simulink model "air_part1_python"  (R2022b)
settings: Solver=FixedStepAuto  StartTime=0.0  StopTime=35  FixedStep=0.00005  MinStep=1e-3  RelTol=1e-3
libraries: slrealtimeseriallib x7, simulink x2, instrumentlib x2, etargetslib x1
settings Model: Creator=riku3  LastModifiedBy=riku3
settings SolverCC: ZeroCrossControl=DisableAll  ZeroCrossAlgorithm=Adaptive
settings DebuggingCC: IgnoredZcDiagnostic=none  UnconnectedInputMsg=warning  UnconnectedOutputMsg=warning  UnconnectedLineMsg=warning
settings ModelReferenceCC: EnableRefExpFcnMdlSchedulingChecks=on
settings RTWCC: DLArmComputeVersion=19.05

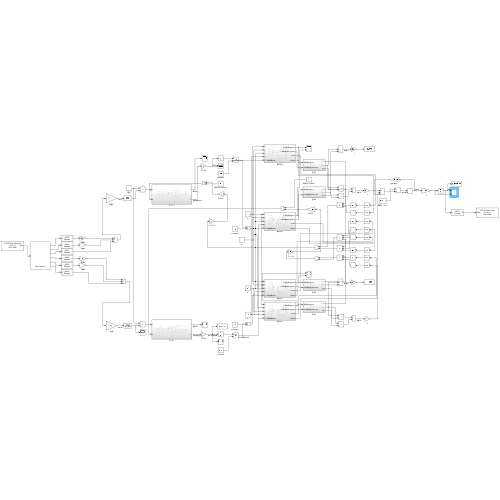
[thumbnail: Simulink's stored preview of the top-level diagram]
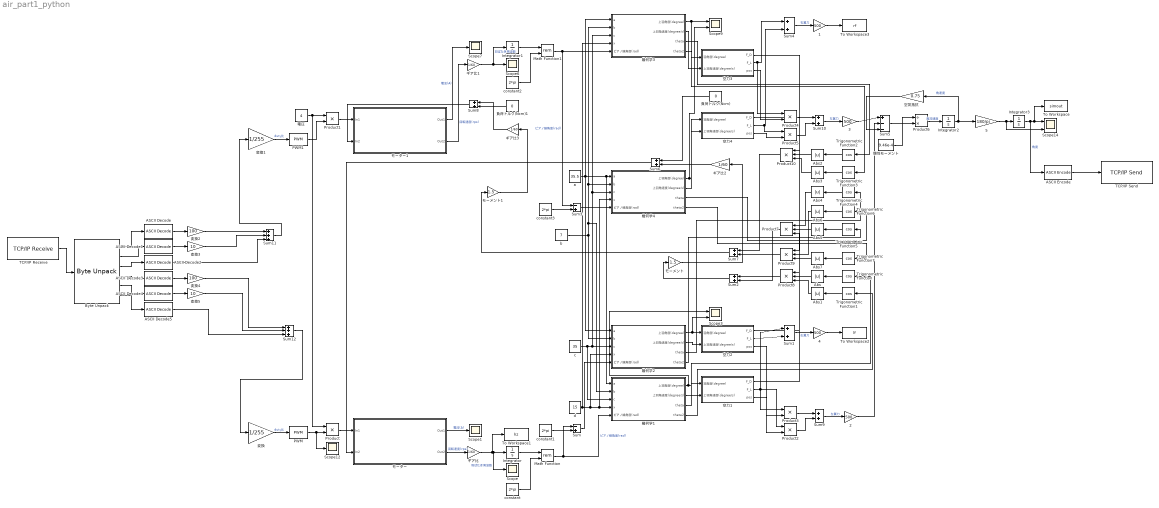
== system air_part1_python ==
  {1..4} (4 alike) : Gain  Gain=500
  5 : Gain  Gain=180/pi
  ASCII Decode{,1..5} (6 alike) : slrealtimeseriallib/ASCII Decode  format=%d\r  nvars=1  vartypes={ }
  ASCII Encode : slrealtimeseriallib/ASCII Encode  format=%d\r  nvars=1  maxlength=128  vartypes={ 'double' }
  Abs{,1..7} (8 alike) : Abs  SaturateOnIntegerOverflow=off
  Byte Unpack : etargetslib/Byte Unpack  dimensions={[1],[1],[1],[1],[1],[1]}  datatypes={'uint8','uint8','uint8','uint8','uint8','uint8'}  byteAlign=1
  Integrator : Integrator
  Integrator1 : Integrator
  Integrator2 : Integrator
  Integrator3 : Integrator  InitialCondition=-90
  Math Function : Math  Operator=rem
  Math Function1 : Math  Operator=rem
  PWM : simulink/Discontinuities/PWM  DisableCoverage=on  Period=0.001  InitialDelay=0  DisallowZeroDutyCycle=off  RunAtFixedTimeIntervals=on  SampleTime=0.00005
  PWM1 : simulink/Discontinuities/PWM  DisableCoverage=on  Period=0.001  InitialDelay=0  DisallowZeroDutyCycle=off  RunAtFixedTimeIntervals=on  SampleTime=0.00005
  Product : Product  Inputs=**
  Product1 : Product  Inputs=**
  Product{7..10} (4 alike) : Product  Inputs=3
  Product{2..5} (4 alike) : Product
  Product6 : Product  Inputs=/*
  Scope{,1,6..7,12} (5 alike) : Scope
  Scope14 : Scope  NumInputPorts=2
  Scope3 : Scope  NumInputPorts=2
  Scope9 : Scope  NumInputPorts=2
  Sum : Sum  Inputs=-+
  Sum1 : Sum  Inputs=|++
  Sum{2,6..10} (6 alike) : Sum
  Sum11 : Sum  Inputs=+++
  Sum12 : Sum  Inputs=+++
  Sum3 : Sum  Inputs=-+
  Sum4 : Sum  Inputs=|++
  Sum5 : Sum  Inputs=|+--
  TCP/IP Receive : instrumentlib/TCP//IP Receive  Host=127.0.0.1  Port=9999  DataSize=[6]  DataType=uint8  ASCIIFormatting=%d  Terminator=LF  CustomTerminator=10  ByteOrder=big-endian  EnableBlockingMode=on  Timeout=10  SampleTime=0.04  SimulateUsing=Interpreted execution
  TCP/IP Send : instrumentlib/TCP//IP Send  Host=127.0.0.1  Port=9999  ByteOrder=big-endian  EnableBlockingMode=on  Timeout=10  TransferDelay=on  SimulateUsing=Interpreted execution
  To Workspace : ToWorkspace  VariableName=simout  SaveFormat=Timeseries  SampleTime=-1
  To Workspace1 : ToWorkspace  VariableName=hz  SaveFormat=Timeseries  SampleTime=-1
  To Workspace2 : ToWorkspace  VariableName=lf  SaveFormat=Timeseries  SampleTime=-1
  To Workspace3 : ToWorkspace  VariableName=rf  SaveFormat=Timeseries  SampleTime=-1
  Trigonometric Function{,1..7} (8 alike) : Trigonometry  Operator=cos
  a : Constant  Value=35.5
  b : Constant  Value=7
  c : Constant  Value=35
  constant{,1..3} (4 alike) : Constant  Value=2*pi
  d : Constant  Value=15
  ギア比{,1..3} (4 alike) : Gain  Gain=1/60
  モーター : Subsystem
  モーター1 : Subsystem
  モーメント : Gain  Gain=1.5
  モーメント1 : Gain  Gain=1.5
  変換 : Gain  Gain=1/255
  変換1 : Gain  Gain=1/255
  変換2 : Gain  Gain=100
  変換3 : Gain  Gain=10
  変換4 : Gain  Gain=100
  変換5 : Gain  Gain=10
  幾何学1 : Subsystem
  幾何学2 : Subsystem
  幾何学3 : Subsystem
  幾何学4 : Subsystem
  慣性モーメント : Constant  Value=9.46e-4
  空力1 : Subsystem
  空力2 : Subsystem
  空力3 : Subsystem
  空力4 : Subsystem
  空気抵抗 : Gain  Gain=0.75
  負荷トルク(Ncm) : Constant  Value=0
  負荷トルク(Ncm)1 : Constant  Value=0
  電圧 : Constant  Value=4
  wires:
  空力2/1(F_D) -> Product7/3
  Abs1/1 -> Product8/3
  Byte Unpack/1 -> ASCII Decode/1
  Byte Unpack/4 -> ASCII Decode3/1
  変換/1 -> PWM/1  "duty比"
  Product1/1 -> モーター1/1(In1)
  変換1/1 -> PWM1/1  "duty比"
  電圧/1 -> Product/1, Product1/1
  PWM1/1 -> Product1/2
  Sum2/1 -> モーメント/1
  PWM/1 -> Scope12/1, Product/2
  Product/1 -> モーター/1(In1)
  ギア比2/1 -> Sum6/2
  モーター1/1(Out1) -> Scope7/1  "電流(A)"
  幾何学1/3(theta) -> Trigonometric Function/1
  幾何学4/3(theta) -> Trigonometric Function6/1
  モーター1/2(Out2) -> ギア比1/1  "回転速度(rps)"
  モーター/2(Out2) -> ギア比/1  "回転速度(rps)"
  モーター/1(Out1) -> Scope1/1  "電流(A)"
  Sum8/1 -> モーター1/2(In2)
  ギア比3/1 -> Sum8/1
  ギア比1/1 -> Integrator1/1, Scope6/1  "羽ばたき周波数"
  Abs2/1 -> Product10/2
  幾何学3/4(theta2) -> Trigonometric Function3/1
  モーメント1/1 -> ギア比3/1
  Sum5/1 -> Product6/2
  空力4/2(F_L) -> Sum4/2, Product5/1
  幾何学2/4(theta2) -> Trigonometric Function5/1
  ギア比/1 -> Integrator/1, Scope/1, To Workspace1/1  "羽ばたき周波数"
  負荷トルク(Ncm)1/1 -> Sum8/2
  Integrator1/1 -> Math Function1/1
  幾何学1/4(theta2) -> Trigonometric Function1/1
  constant2/1 -> Math Function1/2
  Integrator/1 -> Math Function/1
  constant/1 -> Math Function/2
  Math Function1/1 -> Sum3/1, 幾何学3/5(ピアノ線角度(rad))  "ピアノ線角度(rad)"
  空力3/2(F_L) -> Sum4/1, Product4/1
  constant3/1 -> Sum3/2
  constant1/1 -> Sum/2
  幾何学3/2(上羽角速度(degree/s)) -> 空力3/2(上羽角速度(degree/s))
  Math Function/1 -> 幾何学1/5(ピアノ線角度(rad)), Sum/1  "ピアノ線角度(rad)"
  幾何学1/1(上羽角度(degree)) -> Scope3/1, 空力1/1(羽角度(degree))
  Sum3/1 -> 幾何学4/5(ピアノ線角度(rad))
  幾何学4/2(上羽角速度(degree/s)) -> 空力4/2(上羽角速度(degree/s))
  a/1 -> 幾何学1/1(a), 幾何学4/1(a), 幾何学3/1(a), 幾何学2/1(a)
  空力4/3(pos) -> Product5/2
  b/1 -> 幾何学3/2(b), 幾何学4/2(b), 幾何学1/2(b), 幾何学2/2(b)
  空力3/3(pos) -> Product4/2
  c/1 -> 幾何学4/3(c), 幾何学3/3(c), 幾何学2/3(c), 幾何学1/3(c)
  空力4/1(F_D) -> Product9/1
  d/1 -> 幾何学1/4(x), 幾何学4/4(x), 幾何学2/4(x), 幾何学3/4(x)
  Sum/1 -> 幾何学2/5(ピアノ線角度(rad))
  Sum6/1 -> モーター/2(In2)
  空力3/1(F_D) -> Product10/1
  幾何学3/1(上羽角度(degree)) -> Scope9/1, 空力3/1(羽角度(degree))
  空力2/3(pos) -> Product2/2
  幾何学3/3(theta) -> Trigonometric Function2/1
  幾何学4/1(上羽角度(degree)) -> Scope9/2, 空力4/1(羽角度(degree))
  幾何学4/4(theta2) -> Trigonometric Function7/1
  5/1 -> Scope14/2, Integrator3/1
  モーメント/1 -> ギア比2/1
  幾何学2/1(上羽角度(degree)) -> Scope3/2, 空力2/1(羽角度(degree))
  幾何学2/2(上羽角速度(degree/s)) -> 空力2/2(上羽角速度(degree/s))
  幾何学2/3(theta) -> Trigonometric Function4/1
  負荷トルク(Ncm)/1 -> Sum6/1
  幾何学1/2(上羽角速度(degree/s)) -> 空力1/2(上羽角速度(degree/s))
  Sum7/1 -> モーメント1/1
  空力2/2(F_L) -> Sum1/2
  空力1/1(F_D) -> Product8/1
  Trigonometric Function3/1 -> Abs3/1
  空力1/2(F_L) -> Product2/1, Product3/1, Sum1/1
  空力1/3(pos) -> Product3/2
  Product10/1 -> Sum7/1
  Product7/1 -> Sum2/2
  Product9/1 -> Sum7/2
  Product8/1 -> Sum2/1
  Sum4/1 -> 1/1  "右翼力"
  Product4/1 -> Sum10/1
  Product5/1 -> Sum10/2
  Sum1/1 -> 4/1  "左翼力"
  Product3/1 -> Sum9/1
  Product2/1 -> Sum9/2
  Abs3/1 -> Product10/3
  Abs4/1 -> Product7/1
  Abs6/1 -> Product9/2
  Abs5/1 -> Product7/2
  Abs7/1 -> Product9/3
  Abs/1 -> Product8/2
  1/1 -> To Workspace3/1
  Sum10/1 -> 3/1  "左翼力"
  4/1 -> To Workspace2/1
  Sum9/1 -> 2/1  "左翼力"
  Trigonometric Function2/1 -> Abs2/1
  Trigonometric Function4/1 -> Abs4/1
  Trigonometric Function6/1 -> Abs6/1
  Trigonometric Function5/1 -> Abs5/1
  Trigonometric Function7/1 -> Abs7/1
  Trigonometric Function/1 -> Abs/1
  Trigonometric Function1/1 -> Abs1/1
  3/1 -> Sum5/1
  2/1 -> Sum5/2
  慣性モーメント/1 -> Product6/1
  空気抵抗/1 -> Sum5/3
  Product6/1 -> Integrator2/1  "角加速度"
  Integrator2/1 -> 空気抵抗/1, 5/1  "角速度"
  Integrator3/1 -> ASCII Encode/1, To Workspace/1, Scope14/1  "角度"
  Byte Unpack/3 -> ASCII Decode2/1
  Byte Unpack/2 -> ASCII Decode1/1
  TCP/IP Receive/1 -> Byte Unpack/1
  ASCII Encode/1 -> TCP/IP Send/1
  Byte Unpack/5 -> ASCII Decode4/1
  Byte Unpack/6 -> ASCII Decode5/1
  Sum12/1 -> 変換/1
  Sum11/1 -> 変換1/1
  ASCII Decode/1 -> 変換2/1
  ASCII Decode1/1 -> 変換3/1
  ASCII Decode2/1 -> Sum11/3
  ASCII Decode3/1 -> 変換4/1
  ASCII Decode4/1 -> 変換5/1
  ASCII Decode5/1 -> Sum12/3
  変換3/1 -> Sum11/2
  変換4/1 -> Sum12/1
  変換5/1 -> Sum12/2
  変換2/1 -> Sum11/1

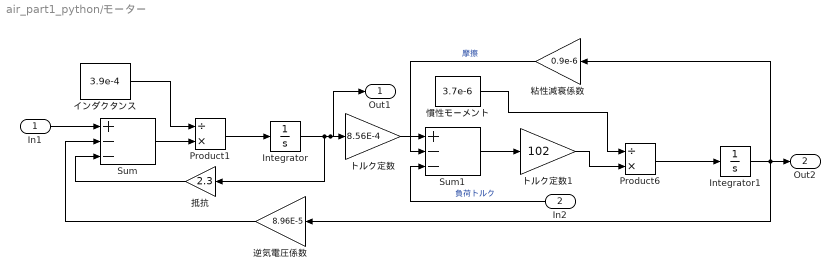
== system air_part1_python/モーター ==
  In1 : Inport
  In2 : Inport  Port=2
  Integrator : Integrator
  Integrator1 : Integrator
  Product1 : Product  Inputs=/*
  Product6 : Product  Inputs=/*
  Sum : Sum  Inputs=+--
  Sum1 : Sum  Inputs=+--
  インダクタンス : Constant  Value=3.9e-4
  トルク定数 : Gain  Gain=8.56E-4
  トルク定数1 : Gain  Gain=102
  慣性モーメント : Constant  Value=3.7e-6
  抵抗 : Gain  Gain=2.3
  粘性減衰係数 : Gain  Gain=0.9e-6
  逆気電圧係数 : Gain  Gain=8.96E-5
  Out1 : Outport
  Out2 : Outport  Port=2
  wires:
  慣性モーメント/1 -> Product6/1
  トルク定数/1 -> Sum1/1
  粘性減衰係数/1 -> Sum1/2  "摩擦"
  In2/1 -> Sum1/3  "負荷トルク"
  抵抗/1 -> Sum/3
  逆気電圧係数/1 -> Sum/2
  In1/1 -> Sum/1
  Product1/1 -> Integrator/1
  インダクタンス/1 -> Product1/1
  Sum/1 -> Product1/2
  Product6/1 -> Integrator1/1
  Integrator1/1 -> 逆気電圧係数/1, 粘性減衰係数/1, Out2/1
  Integrator/1 -> Out1/1, トルク定数/1, 抵抗/1
  Sum1/1 -> トルク定数1/1
  トルク定数1/1 -> Product6/2

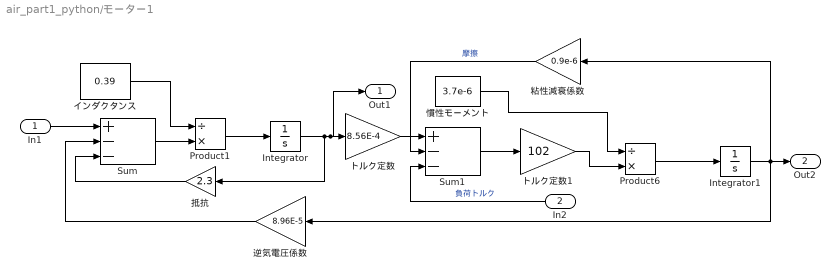
== system air_part1_python/モーター1 ==
  In1 : Inport
  In2 : Inport  Port=2
  Integrator : Integrator
  Integrator1 : Integrator
  Product1 : Product  Inputs=/*
  Product6 : Product  Inputs=/*
  Sum : Sum  Inputs=+--
  Sum1 : Sum  Inputs=+--
  インダクタンス : Constant  Value=0.39
  トルク定数 : Gain  Gain=8.56E-4
  トルク定数1 : Gain  Gain=102
  慣性モーメント : Constant  Value=3.7e-6
  抵抗 : Gain  Gain=2.3
  粘性減衰係数 : Gain  Gain=0.9e-6
  逆気電圧係数 : Gain  Gain=8.96E-5
  Out1 : Outport
  Out2 : Outport  Port=2
  wires:
  慣性モーメント/1 -> Product6/1
  トルク定数/1 -> Sum1/1
  粘性減衰係数/1 -> Sum1/2  "摩擦"
  In2/1 -> Sum1/3  "負荷トルク"
  抵抗/1 -> Sum/3
  逆気電圧係数/1 -> Sum/2
  In1/1 -> Sum/1
  Product1/1 -> Integrator/1
  インダクタンス/1 -> Product1/1
  Sum/1 -> Product1/2
  Product6/1 -> Integrator1/1
  Integrator1/1 -> 逆気電圧係数/1, 粘性減衰係数/1, Out2/1
  Integrator/1 -> Out1/1, トルク定数/1, 抵抗/1
  Sum1/1 -> トルク定数1/1
  トルク定数1/1 -> Product6/2

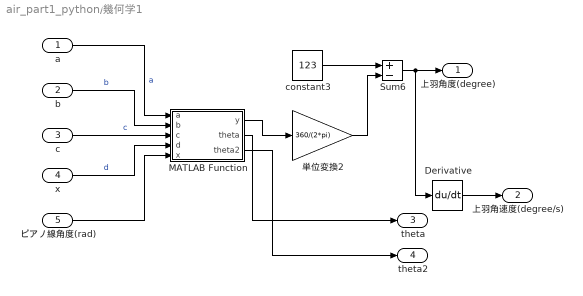
== system air_part1_python/幾何学1 ==
  a : Inport
  b : Inport  Port=2
  c : Inport  Port=3
  x : Inport  Port=4
  ピアノ線角度(rad) : Inport  Port=5
  Derivative : Derivative
  MATLAB Function : MATLAB Function  TreatAsAtomicUnit=on
  Sum6 : Sum  Inputs=+-
  constant3 : Constant  Value=123
  単位変換2 : Gain  Gain=360/(2*pi)
  上羽角度(degree) : Outport
  上羽角速度(degree/s) : Outport  Port=2
  theta : Outport  Port=3
  theta2 : Outport  Port=4
  wires:
  MATLAB Function/1(y) -> 単位変換2/1
  Sum6/1 -> Derivative/1, 上羽角度(degree)/1
  単位変換2/1 -> Sum6/2
  a/1 -> MATLAB Function/1(a)  "a"
  c/1 -> MATLAB Function/3(c)  "c"
  constant3/1 -> Sum6/1
  x/1 -> MATLAB Function/4(d)  "d"
  b/1 -> MATLAB Function/2(b)  "b"
  ピアノ線角度(rad)/1 -> MATLAB Function/5(x)
  Derivative/1 -> 上羽角速度(degree/s)/1
  MATLAB Function/2(theta) -> theta/1
  MATLAB Function/3(theta2) -> theta2/1

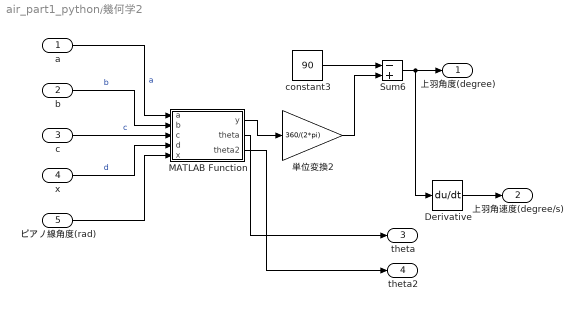
== system air_part1_python/幾何学2 ==
  a : Inport
  b : Inport  Port=2
  c : Inport  Port=3
  x : Inport  Port=4
  ピアノ線角度(rad) : Inport  Port=5
  Derivative : Derivative
  MATLAB Function : MATLAB Function  TreatAsAtomicUnit=on
  Sum6 : Sum  Inputs=-+
  constant3 : Constant  Value=90
  単位変換2 : Gain  Gain=360/(2*pi)
  上羽角度(degree) : Outport
  上羽角速度(degree/s) : Outport  Port=2
  theta : Outport  Port=3
  theta2 : Outport  Port=4
  wires:
  MATLAB Function/1(y) -> 単位変換2/1
  Sum6/1 -> Derivative/1, 上羽角度(degree)/1
  単位変換2/1 -> Sum6/2
  a/1 -> MATLAB Function/1(a)  "a"
  c/1 -> MATLAB Function/3(c)  "c"
  constant3/1 -> Sum6/1
  x/1 -> MATLAB Function/4(d)  "d"
  b/1 -> MATLAB Function/2(b)  "b"
  ピアノ線角度(rad)/1 -> MATLAB Function/5(x)
  Derivative/1 -> 上羽角速度(degree/s)/1
  MATLAB Function/2(theta) -> theta/1
  MATLAB Function/3(theta2) -> theta2/1

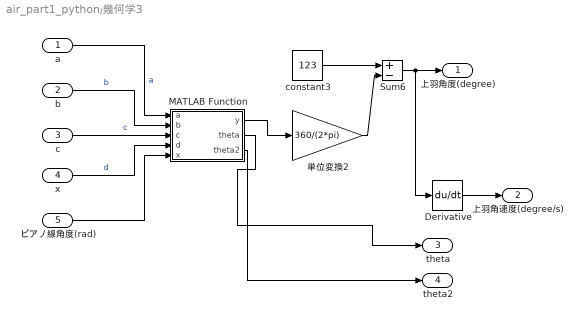
== system air_part1_python/幾何学3 ==
  a : Inport
  b : Inport  Port=2
  c : Inport  Port=3
  x : Inport  Port=4
  ピアノ線角度(rad) : Inport  Port=5
  Derivative : Derivative
  MATLAB Function : MATLAB Function  TreatAsAtomicUnit=on
  Sum6 : Sum  Inputs=+-
  constant3 : Constant  Value=123
  単位変換2 : Gain  Gain=360/(2*pi)
  上羽角度(degree) : Outport
  上羽角速度(degree/s) : Outport  Port=2
  theta : Outport  Port=3
  theta2 : Outport  Port=4
  wires:
  MATLAB Function/1(y) -> 単位変換2/1
  Sum6/1 -> Derivative/1, 上羽角度(degree)/1
  単位変換2/1 -> Sum6/2
  a/1 -> MATLAB Function/1(a)  "a"
  c/1 -> MATLAB Function/3(c)  "c"
  constant3/1 -> Sum6/1
  x/1 -> MATLAB Function/4(d)  "d"
  b/1 -> MATLAB Function/2(b)  "b"
  ピアノ線角度(rad)/1 -> MATLAB Function/5(x)
  Derivative/1 -> 上羽角速度(degree/s)/1
  MATLAB Function/2(theta) -> theta/1
  MATLAB Function/3(theta2) -> theta2/1

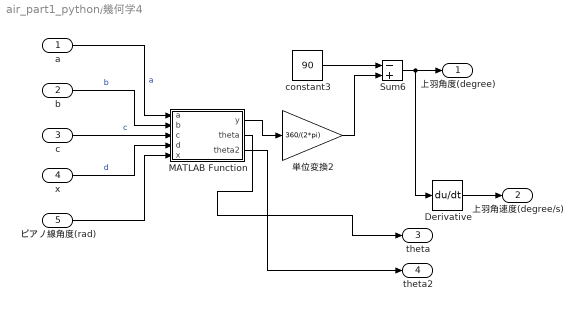
== system air_part1_python/幾何学4 ==
  a : Inport
  b : Inport  Port=2
  c : Inport  Port=3
  x : Inport  Port=4
  ピアノ線角度(rad) : Inport  Port=5
  Derivative : Derivative
  MATLAB Function : MATLAB Function  TreatAsAtomicUnit=on
  Sum6 : Sum  Inputs=-+
  constant3 : Constant  Value=90
  単位変換2 : Gain  Gain=360/(2*pi)
  上羽角度(degree) : Outport
  上羽角速度(degree/s) : Outport  Port=2
  theta : Outport  Port=3
  theta2 : Outport  Port=4
  wires:
  MATLAB Function/1(y) -> 単位変換2/1
  Sum6/1 -> Derivative/1, 上羽角度(degree)/1
  単位変換2/1 -> Sum6/2
  a/1 -> MATLAB Function/1(a)  "a"
  c/1 -> MATLAB Function/3(c)  "c"
  constant3/1 -> Sum6/1
  x/1 -> MATLAB Function/4(d)  "d"
  b/1 -> MATLAB Function/2(b)  "b"
  ピアノ線角度(rad)/1 -> MATLAB Function/5(x)
  Derivative/1 -> 上羽角速度(degree/s)/1
  MATLAB Function/2(theta) -> theta/1
  MATLAB Function/3(theta2) -> theta2/1

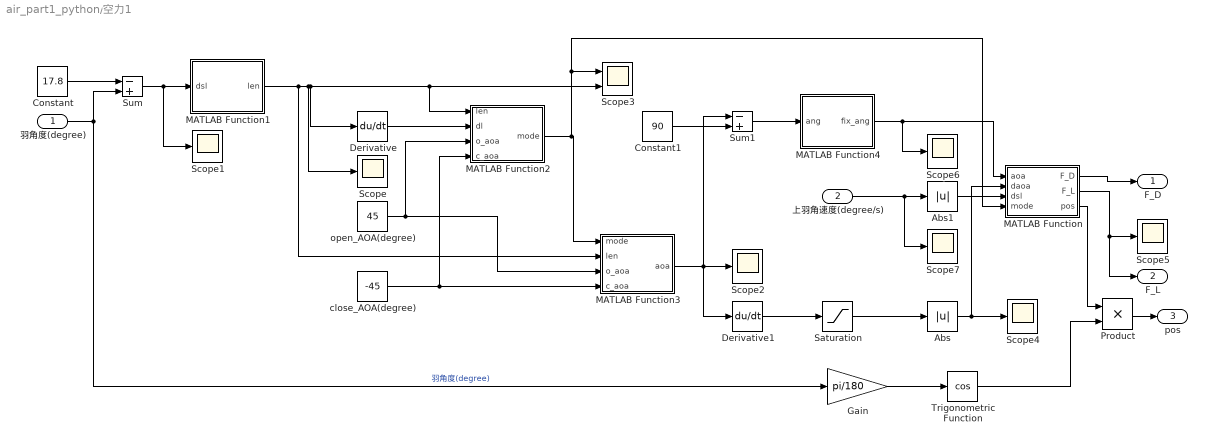
== system air_part1_python/空力1 ==
  羽角度(degree) : Inport
  上羽角速度(degree/s) : Inport  Port=2
  Abs : Abs  SaturateOnIntegerOverflow=off
  Abs1 : Abs  SaturateOnIntegerOverflow=off
  Constant : Constant  Value=17.8
  Constant1 : Constant  Value=90
  Derivative : Derivative
  Derivative1 : Derivative
  Gain : Gain  Gain=pi/180
  MATLAB Function : MATLAB Function  TreatAsAtomicUnit=on
  MATLAB Function1 : MATLAB Function  TreatAsAtomicUnit=on
  MATLAB Function2 : MATLAB Function  TreatAsAtomicUnit=on
  MATLAB Function3 : MATLAB Function  TreatAsAtomicUnit=on
  MATLAB Function4 : MATLAB Function  TreatAsAtomicUnit=on
  Product : Product
  Saturation : Saturate  UpperLimit=5000  LowerLimit=-5000
  Scope{,1..2,4..7} (7 alike) : Scope
  Scope3 : Scope  NumInputPorts=2
  Sum : Sum  Inputs=-+
  Sum1 : Sum  Inputs=-+
  Trigonometric Function : Trigonometry  Operator=cos
  close_AOA(degree) : Constant  Value=-45
  open_AOA(degree) : Constant  Value=45
  F_D : Outport
  F_L : Outport  Port=2
  pos : Outport  Port=3
  wires:
  Constant/1 -> Sum/1
  close_AOA(degree)/1 -> MATLAB Function3/4(c_aoa), MATLAB Function2/4(c_aoa)
  open_AOA(degree)/1 -> MATLAB Function3/3(o_aoa), MATLAB Function2/3(o_aoa)
  Saturation/1 -> Abs/1
  羽角度(degree)/1 -> Gain/1, Sum/2  "羽角度(degree)"
  MATLAB Function2/1(mode) -> MATLAB Function/4(mode), Scope3/1, MATLAB Function3/1(mode)
  Derivative/1 -> MATLAB Function2/2(dl)
  Sum/1 -> Scope1/1, MATLAB Function1/1(dsl)
  MATLAB Function1/1(len) -> Scope3/2, MATLAB Function2/1(len), Derivative/1, Scope/1, MATLAB Function3/2(len)
  Constant1/1 -> Sum1/2
  MATLAB Function3/1(aoa) -> Sum1/1, Derivative1/1, Scope2/1
  Sum1/1 -> MATLAB Function4/1(ang)
  Derivative1/1 -> Saturation/1
  MATLAB Function4/1(fix_ang) -> MATLAB Function/1(aoa), Scope6/1
  上羽角速度(degree/s)/1 -> Scope7/1, Abs1/1
  Abs1/1 -> MATLAB Function/3(dsl)
  Abs/1 -> MATLAB Function/2(daoa), Scope4/1
  MATLAB Function/1(F_D) -> F_D/1
  MATLAB Function/2(F_L) -> F_L/1, Scope5/1
  Product/1 -> pos/1
  Trigonometric Function/1 -> Product/2
  Gain/1 -> Trigonometric Function/1
  MATLAB Function/3(pos) -> Product/1

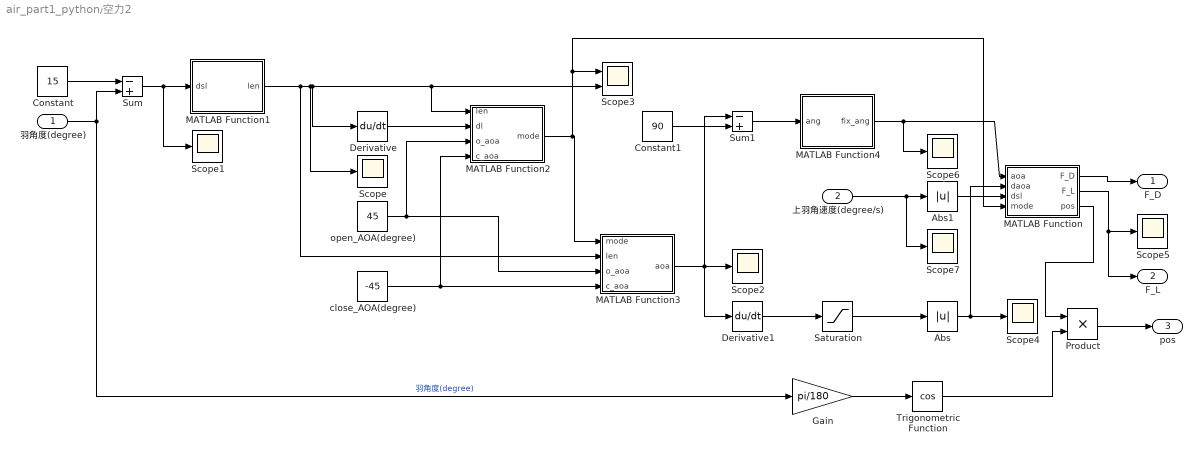
== system air_part1_python/空力2 ==
  羽角度(degree) : Inport
  上羽角速度(degree/s) : Inport  Port=2
  Abs : Abs  SaturateOnIntegerOverflow=off
  Abs1 : Abs  SaturateOnIntegerOverflow=off
  Constant : Constant  Value=15
  Constant1 : Constant  Value=90
  Derivative : Derivative
  Derivative1 : Derivative
  Gain : Gain  Gain=pi/180
  MATLAB Function : MATLAB Function  TreatAsAtomicUnit=on
  MATLAB Function1 : MATLAB Function  TreatAsAtomicUnit=on
  MATLAB Function2 : MATLAB Function  TreatAsAtomicUnit=on
  MATLAB Function3 : MATLAB Function  TreatAsAtomicUnit=on
  MATLAB Function4 : MATLAB Function  TreatAsAtomicUnit=on
  Product : Product
  Saturation : Saturate  UpperLimit=5000  LowerLimit=-5000
  Scope{,1..2,4..7} (7 alike) : Scope
  Scope3 : Scope  NumInputPorts=2
  Sum : Sum  Inputs=-+
  Sum1 : Sum  Inputs=-+
  Trigonometric Function : Trigonometry  Operator=cos
  close_AOA(degree) : Constant  Value=-45
  open_AOA(degree) : Constant  Value=45
  F_D : Outport
  F_L : Outport  Port=2
  pos : Outport  Port=3
  wires:
  Constant/1 -> Sum/1
  close_AOA(degree)/1 -> MATLAB Function3/4(c_aoa), MATLAB Function2/4(c_aoa)
  open_AOA(degree)/1 -> MATLAB Function3/3(o_aoa), MATLAB Function2/3(o_aoa)
  Saturation/1 -> Abs/1
  羽角度(degree)/1 -> Gain/1, Sum/2  "羽角度(degree)"
  MATLAB Function2/1(mode) -> MATLAB Function/4(mode), Scope3/1, MATLAB Function3/1(mode)
  Derivative/1 -> MATLAB Function2/2(dl)
  Sum/1 -> Scope1/1, MATLAB Function1/1(dsl)
  MATLAB Function1/1(len) -> Scope3/2, MATLAB Function2/1(len), Derivative/1, Scope/1, MATLAB Function3/2(len)
  Constant1/1 -> Sum1/2
  MATLAB Function3/1(aoa) -> Sum1/1, Derivative1/1, Scope2/1
  Sum1/1 -> MATLAB Function4/1(ang)
  Derivative1/1 -> Saturation/1
  MATLAB Function4/1(fix_ang) -> MATLAB Function/1(aoa), Scope6/1
  上羽角速度(degree/s)/1 -> Scope7/1, Abs1/1
  Abs1/1 -> MATLAB Function/3(dsl)
  Abs/1 -> MATLAB Function/2(daoa), Scope4/1
  MATLAB Function/1(F_D) -> F_D/1
  MATLAB Function/2(F_L) -> F_L/1, Scope5/1
  Gain/1 -> Trigonometric Function/1
  Trigonometric Function/1 -> Product/2
  Product/1 -> pos/1
  MATLAB Function/3(pos) -> Product/1

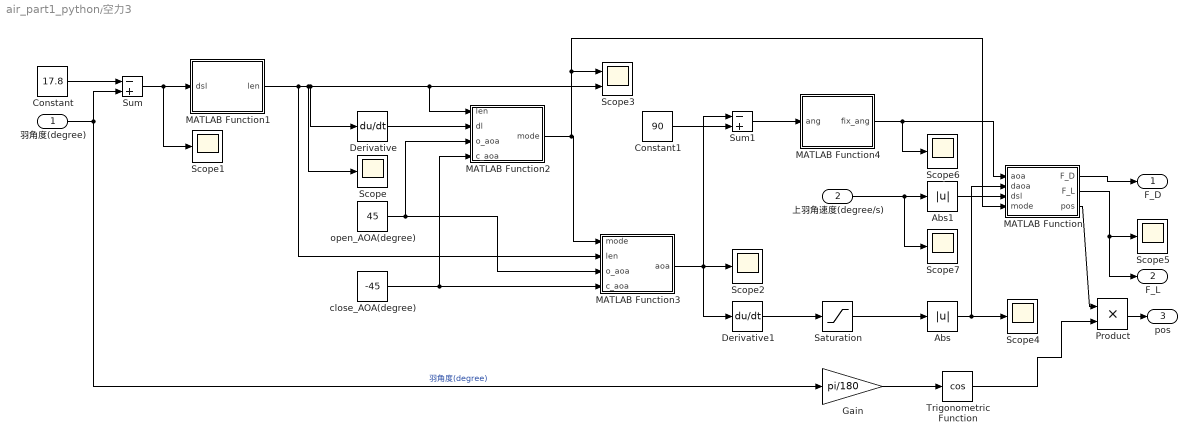
== system air_part1_python/空力3 ==
  羽角度(degree) : Inport
  上羽角速度(degree/s) : Inport  Port=2
  Abs : Abs  SaturateOnIntegerOverflow=off
  Abs1 : Abs  SaturateOnIntegerOverflow=off
  Constant : Constant  Value=17.8
  Constant1 : Constant  Value=90
  Derivative : Derivative
  Derivative1 : Derivative
  Gain : Gain  Gain=pi/180
  MATLAB Function : MATLAB Function  TreatAsAtomicUnit=on
  MATLAB Function1 : MATLAB Function  TreatAsAtomicUnit=on
  MATLAB Function2 : MATLAB Function  TreatAsAtomicUnit=on
  MATLAB Function3 : MATLAB Function  TreatAsAtomicUnit=on
  MATLAB Function4 : MATLAB Function  TreatAsAtomicUnit=on
  Product : Product
  Saturation : Saturate  UpperLimit=5000  LowerLimit=-5000
  Scope{,1..2,4..7} (7 alike) : Scope
  Scope3 : Scope  NumInputPorts=2
  Sum : Sum  Inputs=-+
  Sum1 : Sum  Inputs=-+
  Trigonometric Function : Trigonometry  Operator=cos
  close_AOA(degree) : Constant  Value=-45
  open_AOA(degree) : Constant  Value=45
  F_D : Outport
  F_L : Outport  Port=2
  pos : Outport  Port=3
  wires:
  Constant/1 -> Sum/1
  close_AOA(degree)/1 -> MATLAB Function3/4(c_aoa), MATLAB Function2/4(c_aoa)
  open_AOA(degree)/1 -> MATLAB Function3/3(o_aoa), MATLAB Function2/3(o_aoa)
  Saturation/1 -> Abs/1
  羽角度(degree)/1 -> Sum/2, Gain/1  "羽角度(degree)"
  MATLAB Function2/1(mode) -> MATLAB Function/4(mode), Scope3/1, MATLAB Function3/1(mode)
  Derivative/1 -> MATLAB Function2/2(dl)
  Sum/1 -> Scope1/1, MATLAB Function1/1(dsl)
  MATLAB Function1/1(len) -> Scope3/2, MATLAB Function2/1(len), Derivative/1, Scope/1, MATLAB Function3/2(len)
  Constant1/1 -> Sum1/2
  MATLAB Function3/1(aoa) -> Sum1/1, Derivative1/1, Scope2/1
  Sum1/1 -> MATLAB Function4/1(ang)
  Derivative1/1 -> Saturation/1
  MATLAB Function4/1(fix_ang) -> MATLAB Function/1(aoa), Scope6/1
  上羽角速度(degree/s)/1 -> Scope7/1, Abs1/1
  Abs1/1 -> MATLAB Function/3(dsl)
  Abs/1 -> MATLAB Function/2(daoa), Scope4/1
  MATLAB Function/1(F_D) -> F_D/1
  MATLAB Function/2(F_L) -> F_L/1, Scope5/1
  Gain/1 -> Trigonometric Function/1
  Trigonometric Function/1 -> Product/2
  Product/1 -> pos/1
  MATLAB Function/3(pos) -> Product/1

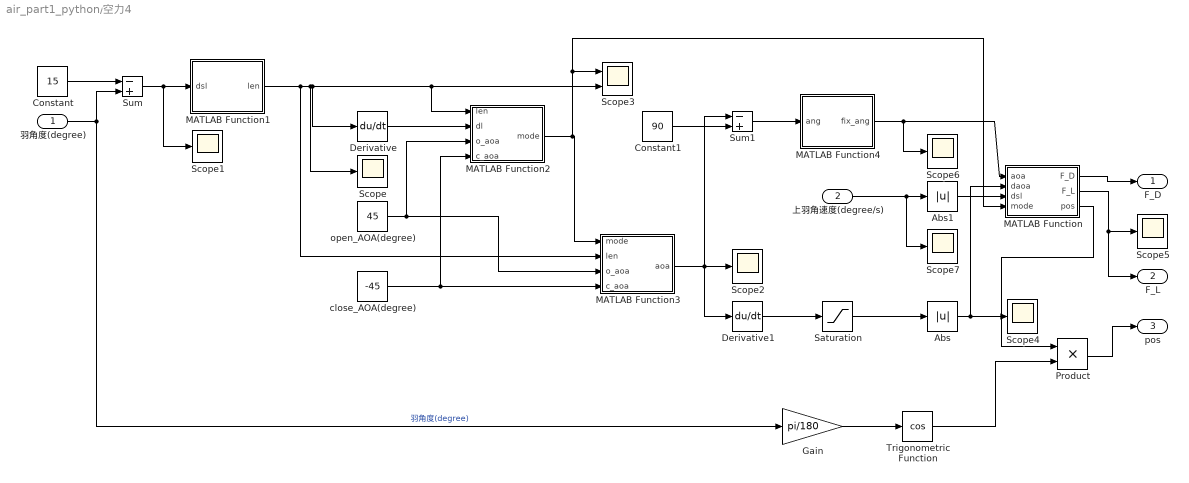
== system air_part1_python/空力4 ==
  羽角度(degree) : Inport
  上羽角速度(degree/s) : Inport  Port=2
  Abs : Abs  SaturateOnIntegerOverflow=off
  Abs1 : Abs  SaturateOnIntegerOverflow=off
  Constant : Constant  Value=15
  Constant1 : Constant  Value=90
  Derivative : Derivative
  Derivative1 : Derivative
  Gain : Gain  Gain=pi/180
  MATLAB Function : MATLAB Function  TreatAsAtomicUnit=on
  MATLAB Function1 : MATLAB Function  TreatAsAtomicUnit=on
  MATLAB Function2 : MATLAB Function  TreatAsAtomicUnit=on
  MATLAB Function3 : MATLAB Function  TreatAsAtomicUnit=on
  MATLAB Function4 : MATLAB Function  TreatAsAtomicUnit=on
  Product : Product
  Saturation : Saturate  UpperLimit=5000  LowerLimit=-5000
  Scope{,1..2,4..7} (7 alike) : Scope
  Scope3 : Scope  NumInputPorts=2
  Sum : Sum  Inputs=-+
  Sum1 : Sum  Inputs=-+
  Trigonometric Function : Trigonometry  Operator=cos
  close_AOA(degree) : Constant  Value=-45
  open_AOA(degree) : Constant  Value=45
  F_D : Outport
  F_L : Outport  Port=2
  pos : Outport  Port=3
  wires:
  Constant/1 -> Sum/1
  close_AOA(degree)/1 -> MATLAB Function3/4(c_aoa), MATLAB Function2/4(c_aoa)
  open_AOA(degree)/1 -> MATLAB Function3/3(o_aoa), MATLAB Function2/3(o_aoa)
  Saturation/1 -> Abs/1
  羽角度(degree)/1 -> Gain/1, Sum/2  "羽角度(degree)"
  MATLAB Function2/1(mode) -> MATLAB Function/4(mode), Scope3/1, MATLAB Function3/1(mode)
  Derivative/1 -> MATLAB Function2/2(dl)
  Sum/1 -> Scope1/1, MATLAB Function1/1(dsl)
  MATLAB Function1/1(len) -> Scope3/2, MATLAB Function2/1(len), Derivative/1, Scope/1, MATLAB Function3/2(len)
  Constant1/1 -> Sum1/2
  MATLAB Function3/1(aoa) -> Sum1/1, Derivative1/1, Scope2/1
  Sum1/1 -> MATLAB Function4/1(ang)
  Derivative1/1 -> Saturation/1
  MATLAB Function4/1(fix_ang) -> MATLAB Function/1(aoa), Scope6/1
  上羽角速度(degree/s)/1 -> Scope7/1, Abs1/1
  Abs1/1 -> MATLAB Function/3(dsl)
  Abs/1 -> MATLAB Function/2(daoa), Scope4/1
  MATLAB Function/1(F_D) -> F_D/1
  MATLAB Function/2(F_L) -> F_L/1, Scope5/1
  Gain/1 -> Trigonometric Function/1
  Trigonometric Function/1 -> Product/2
  Product/1 -> pos/1
  MATLAB Function/3(pos) -> Product/1

== matlab function air_part1_python/空力2/MATLAB Function4 ==
  data: fix_ang output; ang input
function fix_ang = fcn(ang)

if(ang>90)
    fix_ang = 180-ang;
else
    fix_ang = ang;

end

== matlab function air_part1_python/空力1/MATLAB Function ==
  data: aoa input; daoa input; F_D output; dsl input; F_L output; mode input; pos output
function [F_D,F_L,pos]= fcn(aoa,daoa,dsl,mode) %aoa:AOA(degree) daoa:AOA(degree/s) dsl:ストローク角(degree/s)

a = aoa*pi/180;
da = daoa*pi/180;
s = dsl*pi/180;

air = 1.293;    %空気密度 kg/m3
Aw = 0.104;         %翼面積 m3
L = 0.22;       %翼長 m
cm = 0.15;      %最大翼幅 m
r2 = 0.625;       %正規化された圧力中心 0.6-0.7 {S[0->L]c(r)r^2dr}/{L^2Aw} %分子:0.000313609 分母:0.00501908
c_ = 0.1;       %正規化された回転弦 0.5-0.75 {S[0->L]c^2(r)rdr}/{r2LAwcm} %分子:0.00027225 分母:0.002713

Cn = 3.4*sin(a);
if(aoa>45)
    Ct = 0;
else
    Ct = 0.4*(cos(2*a))^2;
end
%Cl = Cn*cos(a)-Ct*sin(a);
%Cd = Cn*sin(a)+Ct*cos(a);
Crot = 2*pi*(3/4-1/4);

Ucp = r2*L*s;
if(mode==1 || mode==3)
    Ftr_N = 1/2*air*Aw*Cn*Ucp^2;
    Ftr_T = 1/2*air*Aw*Ct*Ucp^2;
else
    Ftr_N = 0;
    Ftr_T = 0;
end
Frot_N = 1/2*air*Aw*Crot*c_*cm*da*Ucp;

F_N = Ftr_N+Frot_N;
F_T = Ftr_T;

F_D = F_N*cos(a)-F_T*sin(a);
F_L = F_N*sin(a)+F_T*cos(a);
pos = L*r2;
end

== matlab function air_part1_python/空力1/MATLAB Function1 ==
  data: len output; dsl input
function len = fcn(dsl) %dsl:ストローク角(degree/s)

s = dsl*pi/180;

L = 0.22;       %翼長 m
r2 = 0.625;       %正規化された圧力中心 0.6-0.7 {S[0->L]c(r)r^2dr}/{L^2Aw}

len = L*r2*tan(s);
end

== matlab function air_part1_python/空力1/MATLAB Function2 ==
  data: mode output; len input; dl input; o_aoa input; c_aoa input
function mode = fcn(len,dl,o_aoa,c_aoa)

o = o_aoa*pi/180;
c = -1*c_aoa*pi/180;

wing = 0.1;
ol = wing*sin(o);
cl = wing*sin(c);

if (dl>0 && len>ol)
    mode = 1;
elseif(dl<=0 && len>0.198-2*cl)
    mode = 2;
elseif(dl<=0)
    mode = 3;
else
    mode = 4;
end
end

== matlab function air_part1_python/空力1/MATLAB Function3 ==
  data: aoa output; mode input; len input; o_aoa input; c_aoa input
function aoa = fcn(mode,len,o_aoa,c_aoa)

o = o_aoa*pi/180;
c = -1*c_aoa*pi/180;

wing = 0.1;
h_wing = wing/2;
ol = wing*sin(o);
cl = wing*sin(c);

if(mode==1)
    aoa=o_aoa;
elseif(mode==2)
    aoa=min(asin((ol-(0.198-len))/wing)*180/pi,o_aoa);
    %aoa=0;
elseif(mode==3)
    aoa=c_aoa;
else
    aoa=max(-1*asin((cl/2-len)/h_wing)*180/pi,c_aoa);
    %aoa=0;
end
end

== matlab function air_part1_python/幾何学2/MATLAB Function ==
  data: a input; y output; b input; c input; d input; x input; theta output; theta2 output
function [y,theta,theta2] = fcn(a,b,c,d,x)

h2 = a^2+b^2+2*a*b*cos(x);
h = sqrt(h2);
p = acos((h2+a^2-b^2)/(2*h*a));
q = acos((h2+d^2-c^2)/(2*h*d));

theta = pi/2-acos((-h2+c^2+d^2)/(2*c*d));
theta2 = acos((-d^2+h2+c^2)/(2*h*c));

if x>pi()
    p = -1*p;
    y = p+q;
else
    y = p+q;
end

== matlab function air_part1_python/空力1/MATLAB Function4 ==
  data: fix_ang output; ang input
function fix_ang = fcn(ang)

if(ang>90)
    fix_ang = 180-ang;
else
    fix_ang = ang;

end

== matlab function air_part1_python/空力3/MATLAB Function ==
  data: aoa input; daoa input; F_D output; dsl input; F_L output; mode input; pos output
function [F_D,F_L,pos]= fcn(aoa,daoa,dsl,mode) %aoa:AOA(degree) daoa:AOA(degree/s) dsl:ストローク角(degree/s)

a = aoa*pi/180;
da = daoa*pi/180;
s = dsl*pi/180;

air = 1.293;    %空気密度 kg/m3
Aw = 0.104;         %翼面積 m3
L = 0.22;       %翼長 m
cm = 0.15;      %最大翼幅 m
r2 = 0.625;       %正規化された圧力中心 0.6-0.7 {S[0->L]c(r)r^2dr}/{L^2Aw} %分子:0.000313609 分母:0.00501908
c_ = 0.1;       %正規化された回転弦 0.5-0.75 {S[0->L]c^2(r)rdr}/{r2LAwcm} %分子:0.00027225 分母:0.002713

Cn = 3.4*sin(a);
if(aoa>45)
    Ct = 0;
else
    Ct = 0.4*(cos(2*a))^2;
end
%Cl = Cn*cos(a)-Ct*sin(a);
%Cd = Cn*sin(a)+Ct*cos(a);
Crot = 2*pi*(3/4-1/4);

Ucp = r2*L*s;
if(mode==1 || mode==3)
    Ftr_N = 1/2*air*Aw*Cn*Ucp^2;
    Ftr_T = 1/2*air*Aw*Ct*Ucp^2;
else
    Ftr_N = 0;
    Ftr_T = 0;
end
Frot_N = 1/2*air*Aw*Crot*c_*cm*da*Ucp;

F_N = Ftr_N+Frot_N;
F_T = Ftr_T;

F_D = F_N*cos(a)-F_T*sin(a);
F_L = F_N*sin(a)+F_T*cos(a);
pos = L*r2;
end

== matlab function air_part1_python/空力3/MATLAB Function1 ==
  data: len output; dsl input
function len = fcn(dsl) %dsl:ストローク角(degree/s)

s = dsl*pi/180;

L = 0.22;       %翼長 m
r2 = 0.625;       %正規化された圧力中心 0.6-0.7 {S[0->L]c(r)r^2dr}/{L^2Aw}

len = L*r2*tan(s);
end

== matlab function air_part1_python/空力3/MATLAB Function2 ==
  data: mode output; len input; dl input; o_aoa input; c_aoa input
function mode = fcn(len,dl,o_aoa,c_aoa)

o = o_aoa*pi/180;
c = -1*c_aoa*pi/180;

wing = 0.1;
ol = wing*sin(o);
cl = wing*sin(c);

if (dl>0 && len>ol)
    mode = 1;
elseif(dl<=0 && len>0.198-2*cl)
    mode = 2;
elseif(dl<=0)
    mode = 3;
else
    mode = 4;
end
end

== matlab function air_part1_python/空力3/MATLAB Function3 ==
  data: aoa output; mode input; len input; o_aoa input; c_aoa input
function aoa = fcn(mode,len,o_aoa,c_aoa)

o = o_aoa*pi/180;
c = -1*c_aoa*pi/180;

wing = 0.1;
h_wing = wing/2;
ol = wing*sin(o);
cl = wing*sin(c);

if(mode==1)
    aoa=o_aoa;
elseif(mode==2)
    aoa=min(asin((ol-(0.198-len))/wing)*180/pi,o_aoa);
    %aoa=0;
elseif(mode==3)
    aoa=c_aoa;
else
    aoa=max(-1*asin((cl/2-len)/h_wing)*180/pi,c_aoa);
    %aoa=0;
end
end

== matlab function air_part1_python/空力3/MATLAB Function4 ==
  data: fix_ang output; ang input
function fix_ang = fcn(ang)

if(ang>90)
    fix_ang = 180-ang;
else
    fix_ang = ang;

end

== matlab function air_part1_python/空力4/MATLAB Function ==
  data: aoa input; daoa input; F_D output; dsl input; F_L output; mode input; pos output
function [F_D,F_L,pos]= fcn(aoa,daoa,dsl,mode) %aoa:AOA(degree) daoa:AOA(degree/s) dsl:ストローク角(degree/s)

a = aoa*pi/180;
da = daoa*pi/180;
s = dsl*pi/180;

air = 1.293;    %空気密度 kg/m3
Aw = 0.104;         %翼面積 m3
L = 0.22;       %翼長 m
cm = 0.15;      %最大翼幅 m
r2 = 0.625;       %正規化された圧力中心 0.6-0.7 {S[0->L]c(r)r^2dr}/{L^2Aw} %分子:0.000313609 分母:0.00501908
c_ = 0.1;       %正規化された回転弦 0.5-0.75 {S[0->L]c^2(r)rdr}/{r2LAwcm} %分子:0.00027225 分母:0.002713

Cn = 3.4*sin(a);
if(aoa>45)
    Ct = 0;
else
    Ct = 0.4*(cos(2*a))^2;
end
%Cl = Cn*cos(a)-Ct*sin(a);
%Cd = Cn*sin(a)+Ct*cos(a);
Crot = 2*pi*(3/4-1/4);

Ucp = r2*L*s;
if(mode==1 || mode==3)
    Ftr_N = 1/2*air*Aw*Cn*Ucp^2;
    Ftr_T = 1/2*air*Aw*Ct*Ucp^2;
else
    Ftr_N = 0;
    Ftr_T = 0;
end
Frot_N = 1/2*air*Aw*Crot*c_*cm*da*Ucp;

F_N = Ftr_N+Frot_N;
F_T = Ftr_T;

F_D = F_N*cos(a)-F_T*sin(a);
F_L = F_N*sin(a)+F_T*cos(a);
pos = L*r2;
end

== matlab function air_part1_python/空力4/MATLAB Function1 ==
  data: len output; dsl input
function len = fcn(dsl) %dsl:ストローク角(degree/s)

s = dsl*pi/180;

L = 0.22;       %翼長 m
r2 = 0.625;       %正規化された圧力中心 0.6-0.7 {S[0->L]c(r)r^2dr}/{L^2Aw}

len = L*r2*tan(s);
end

== matlab function air_part1_python/空力4/MATLAB Function2 ==
  data: mode output; len input; dl input; o_aoa input; c_aoa input
function mode = fcn(len,dl,o_aoa,c_aoa)

o = o_aoa*pi/180;
c = -1*c_aoa*pi/180;

wing = 0.1;
ol = -1*wing*sin(o);
cl = -1*wing*sin(c);

if (dl<0 && len<ol)
    mode = 1;
elseif(dl>=0 && len<-0.197-2*cl)
    mode = 2;
elseif(dl>=0)
    mode = 3;
else
    mode = 4;
end
end

== matlab function air_part1_python/空力4/MATLAB Function3 ==
  data: aoa output; mode input; len input; o_aoa input; c_aoa input
function aoa = fcn(mode,len,o_aoa,c_aoa)

o = o_aoa*pi/180;
c = -1*c_aoa*pi/180;

wing = 0.1;
h_wing = wing/2;
ol = wing*sin(o);
cl = wing*sin(c);

if(mode==1)
    aoa=o_aoa;
elseif(mode==2)
    aoa=min(asin((ol-(len+0.197))/wing)*180/pi,o_aoa);
elseif(mode==3)
    aoa=c_aoa;
else
    aoa=max(-1*asin((cl/2+len)/h_wing)*180/pi,c_aoa);
end
end

== matlab function air_part1_python/空力4/MATLAB Function4 ==
  data: fix_ang output; ang input
function fix_ang = fcn(ang)

if(ang>90)
    fix_ang = 180-ang;
else
    fix_ang = ang;

end

== matlab function air_part1_python/幾何学1/MATLAB Function ==
  data: a input; y output; b input; c input; d input; x input; theta output; theta2 output
function [y,theta,theta2] = fcn(a,b,c,d,x)

h2 = a^2+b^2+2*a*b*cos(x);
h = sqrt(h2);
p = acos((h2+a^2-b^2)/(2*h*a));
q = acos((h2+d^2-c^2)/(2*h*d));

theta = pi/2-acos((-h2+c^2+d^2)/(2*c*d));
theta2 = acos((-d^2+h2+c^2)/(2*h*c));

if x>pi()
    p = -1*p;
    y = p+q;
else
    y = p+q;
end

== matlab function air_part1_python/幾何学3/MATLAB Function ==
  data: a input; y output; b input; c input; d input; x input; theta output; theta2 output
function [y,theta,theta2] = fcn(a,b,c,d,x)

h2 = a^2+b^2+2*a*b*cos(x);
h = sqrt(h2);
p = acos((h2+a^2-b^2)/(2*h*a));
q = acos((h2+d^2-c^2)/(2*h*d));

theta = pi/2-acos((-h2+c^2+d^2)/(2*c*d));
theta2 = acos((-d^2+h2+c^2)/(2*h*c));

if x>pi()
    p = -1*p;
    y = p+q;
else
    y = p+q;
end

== matlab function air_part1_python/幾何学4/MATLAB Function ==
  data: a input; y output; b input; c input; d input; x input; theta output; theta2 output
function [y,theta,theta2] = fcn(a,b,c,d,x)

h2 = a^2+b^2+2*a*b*cos(x);
h = sqrt(h2);
p = acos((h2+a^2-b^2)/(2*h*a));
q = acos((h2+d^2-c^2)/(2*h*d));

theta = pi/2-acos((-h2+c^2+d^2)/(2*c*d));
theta2 = acos((-d^2+h2+c^2)/(2*h*c));

if x>pi()
    p = -1*p;
    y = p+q;
else
    y = p+q;
end

== matlab function air_part1_python/空力2/MATLAB Function ==
  data: aoa input; daoa input; F_D output; dsl input; F_L output; mode input; pos output
function [F_D,F_L,pos]= fcn(aoa,daoa,dsl,mode) %aoa:AOA(degree) daoa:AOA(degree/s) dsl:ストローク角(degree/s)

a = aoa*pi/180;
da = daoa*pi/180;
s = dsl*pi/180;

air = 1.293;    %空気密度 kg/m3
Aw = 0.104;         %翼面積 m3
L = 0.22;       %翼長 m
cm = 0.15;      %最大翼幅 m
r2 = 0.625;       %正規化された圧力中心 0.6-0.7 {S[0->L]c(r)r^2dr}/{L^2Aw} %分子:0.000313609 分母:0.00501908
c_ = 0.1;       %正規化された回転弦 0.5-0.75 {S[0->L]c^2(r)rdr}/{r2LAwcm} %分子:0.00027225 分母:0.002713

Cn = 3.4*sin(a);
if(aoa>45)
    Ct = 0;
else
    Ct = 0.4*(cos(2*a))^2;
end
%Cl = Cn*cos(a)-Ct*sin(a);
%Cd = Cn*sin(a)+Ct*cos(a);
Crot = 2*pi*(3/4-1/4);

Ucp = r2*L*s;
if(mode==1 || mode==3)
    Ftr_N = 1/2*air*Aw*Cn*Ucp^2;
    Ftr_T = 1/2*air*Aw*Ct*Ucp^2;
else
    Ftr_N = 0;
    Ftr_T = 0;
end
Frot_N = 1/2*air*Aw*Crot*c_*cm*da*Ucp;

F_N = Ftr_N+Frot_N;
F_T = Ftr_T;

F_D = F_N*cos(a)-F_T*sin(a);
F_L = F_N*sin(a)+F_T*cos(a);
pos = L*r2;
end

== matlab function air_part1_python/空力2/MATLAB Function1 ==
  data: len output; dsl input
function len = fcn(dsl) %dsl:ストローク角(degree/s)

s = dsl*pi/180;

L = 0.22;       %翼長 m
r2 = 0.625;       %正規化された圧力中心 0.6-0.7 {S[0->L]c(r)r^2dr}/{L^2Aw}

len = L*r2*tan(s);
end

== matlab function air_part1_python/空力2/MATLAB Function2 ==
  data: mode output; len input; dl input; o_aoa input; c_aoa input
function mode = fcn(len,dl,o_aoa,c_aoa)

o = o_aoa*pi/180;
c = -1*c_aoa*pi/180;

wing = 0.1;
ol = -1*wing*sin(o);
cl = -1*wing*sin(c);

if (dl<0 && len<ol)
    mode = 1;
elseif(dl>=0 && len<-0.197-2*cl)
    mode = 2;
elseif(dl>=0)
    mode = 3;
else
    mode = 4;
end
end

== matlab function air_part1_python/空力2/MATLAB Function3 ==
  data: aoa output; mode input; len input; o_aoa input; c_aoa input
function aoa = fcn(mode,len,o_aoa,c_aoa)

o = o_aoa*pi/180;
c = -1*c_aoa*pi/180;

wing = 0.1;
h_wing = wing/2;
ol = wing*sin(o);
cl = wing*sin(c);

if(mode==1)
    aoa=o_aoa;
elseif(mode==2)
    aoa=min(asin((ol-(len+0.197))/wing)*180/pi,o_aoa);
elseif(mode==3)
    aoa=c_aoa;
else
    aoa=max(-1*asin((cl/2+len)/h_wing)*180/pi,c_aoa);
end
end
